simulink model "Final"  (R2025b)
settings: Solver=ode4  StartTime=0.0  StopTime=3  FixedStep=1e-5  RelTol=1e-3
values from neighbouring files (symbols this model uses):
  BAT_A = BAT    [simulink_init_params_CORRECTED.m]
  BAT_B = BAT    [simulink_init_params_CORRECTED.m]
  omega_init_cmd = SpeedRef_rpm_cmd * 2 * pi / 60    (= 314.159265359)    [simulink_init_params_CORRECTED.m]
  SpeedRef_rpm_cmd = 3000    [simulink_init_params_CORRECTED.m]
  TorqueRef_gen_Nm_cmd = -100    [simulink_init_params_CORRECTED.m]
undefined symbols (not defined in the file or in its folder): BAT, DCDC, DCLINK, FOC, FW, INV, MECH, PMSM, THERM
libraries: slpidlib x6, mcbcontrolslib x2
(part 2 of 2)

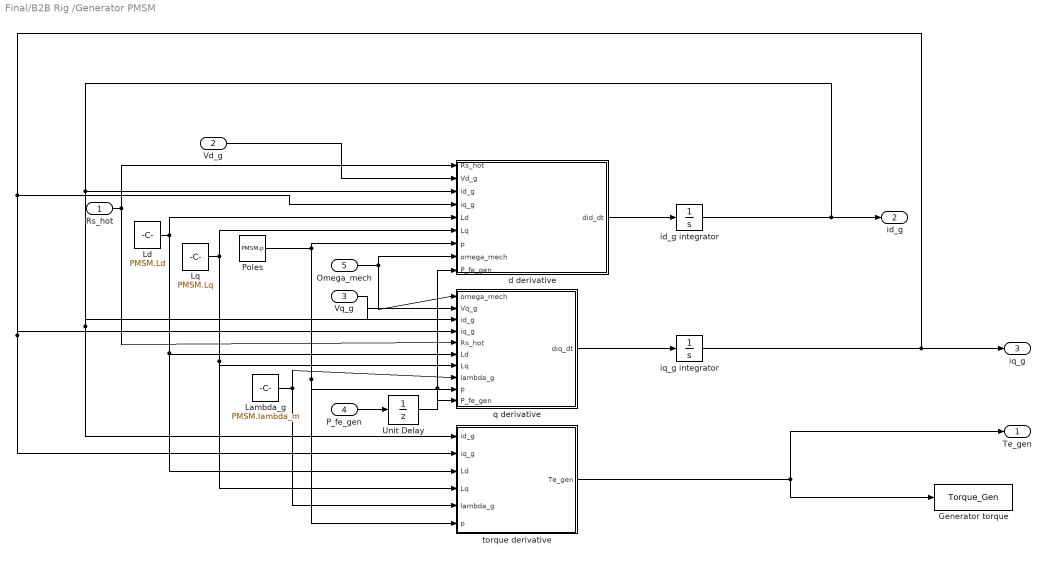
== system Final/B2B Rig /Generator PMSM ==
  Rs_hot : Inport
  Vd_g : Inport  Port=2
  Vq_g : Inport  Port=3
  P_fe_gen : Inport  Port=4
  Omega_mech : Inport  Port=5
  Generator torque : ToWorkspace  VariableName=Torque_Gen  SaveFormat=Timeseries  SampleTime=-1
  Lambda_g : Constant  Value=PMSM.lambda_m
  Ld : Constant  Value=PMSM.Ld
  Lq : Constant  Value=PMSM.Lq
  Poles : Constant  Value=PMSM.p
  Unit Delay : UnitDelay  SampleTime=FOC.Ts  HasFrameUpgradeWarning=on
  d derivative : MATLAB Function  TreatAsAtomicUnit=on
  id_g integrator : Integrator
  iq_g integrator : Integrator
  q derivative : MATLAB Function  TreatAsAtomicUnit=on
  torque derivative : MATLAB Function  TreatAsAtomicUnit=on
  Te_gen : Outport
  id_g : Outport  Port=2
  iq_g : Outport  Port=3
  wires:
  Lq/1 -> torque derivative/4(Lq), q derivative/7(Lq), d derivative/6(Lq)
  Poles/1 -> torque derivative/6(p), q derivative/9(p), d derivative/7(p)
  id_g integrator/1 -> id_g/1, d derivative/3(id_g), torque derivative/1(id_g), q derivative/3(id_g)
  Ld/1 -> torque derivative/3(Ld), q derivative/6(Ld), d derivative/5(Ld)
  iq_g integrator/1 -> iq_g/1, torque derivative/2(iq_g), q derivative/4(iq_g), d derivative/4(iq_g)
  Lambda_g/1 -> q derivative/8(lambda_g), torque derivative/5(lambda_g)
  Rs_hot/1 -> d derivative/1(Rs_hot), q derivative/5(Rs_hot)
  q derivative/1(diq_dt) -> iq_g integrator/1
  Omega_mech/1 -> q derivative/1(omega_mech), d derivative/8(omega_mech)
  Vq_g/1 -> q derivative/2(Vq_g)
  d derivative/1(did_dt) -> id_g integrator/1
  torque derivative/1(Te_gen) -> Generator torque/1, Te_gen/1
  Vd_g/1 -> d derivative/2(Vd_g)
  Unit Delay/1 -> d derivative/9(P_fe_gen), q derivative/10(P_fe_gen)
  P_fe_gen/1 -> Unit Delay/1

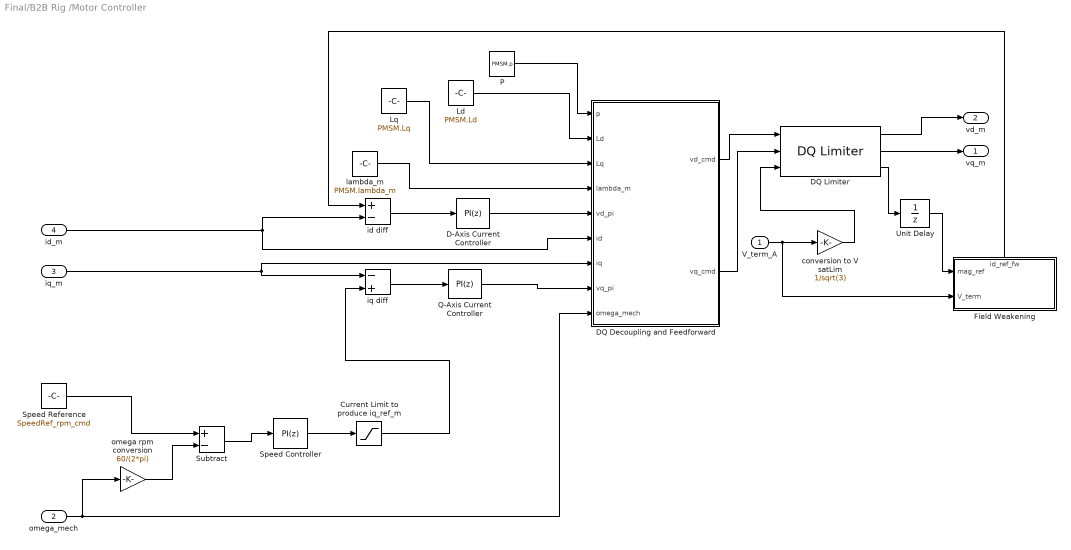
== system Final/B2B Rig /Motor Controller ==
  V_term_A : Inport
  omega_mech : Inport  Port=2
  iq_m : Inport  Port=3
  id_m : Inport  Port=4
  " Speed Controller" : slpidlib/PID Controller  Controller=PI  Form=Parallel  TimeDomain=Discrete-time  UseExternalTs=off  SampleTime=FOC.Ts  IntegratorMethod=Forward Euler  FilterMethod=Forward Euler  ControllerParametersSource=internal  P=FOC.Kp_speed  I=FOC.Ki_speed  UseKiTs=off  D=0  UseExternalDerivativeSource=off  N=100  UseFilter=on  TunerSelectOption=Transfer Function Based (PID Tuner App)  InitialConditionSource=internal  InitialConditionForIntegrator=0  InitialConditionForFilter=0  DifferentiatorICPrevScaledInput=0  ExternalReset=none  TrackingMode=off  Kt=1  LimitOutput=on  SatLimitsSource=internal  UpperSaturationLimit=FOC.I_limit  LowerSaturationLimit=-FOC.I_limit  LinearizeAsGain=on  AntiWindupMode=clamping  Kb=1  LimitIntegrator=off  UpperIntegratorSaturationLimit=inf  LowerIntegratorSaturationLimit=-inf  POutMin=[]  POutMax=[]  IOutMin=[]  IOutMax=[]  DOutMin=[]  DOutMax=[]  NOutMin=[]  NOutMax=[]  SumOutMin=[]  SumOutMax=[]  SaturationOutMin=[]  SaturationOutMax=[]  PParamMin=[]  PParamMax=[]  IParamMin=[]  IParamMax=[]  DParamMin=[]  DParamMax=[]  NParamMin=[]  NParamMax=[]  KbParamMin=[]  KbParamMax=[]  KtParamMin=[]  KtParamMax=[]  KbOutMin=[]  KbOutMax=[]  KtOutMin=[]  KtOutMax=[]  IntegratorOutMin=[]  IntegratorOutMax=[]  FilterOutMin=[]  FilterOutMax=[]  SumI1OutMin=[]  SumI1OutMax=[]  SumI2OutMin=[]  SumI2OutMax=[]  SumI3OutMin=[]  SumI3OutMax=[]  SumI4OutMin=[]  SumI4OutMax=[]  SumDOutMin=[]  SumDOutMax=[]  DifferentiatorOutMin=[]  DifferentiatorOutMax=[]  FilterDiffOutCoefMin=[]  FilterDiffOutCoefMax=[]  ReciprocalOutMin=[]  ReciprocalOutMax=[]  SumDenOutMin=[]  SumDenOutMax=[]  SumNumOutMin=[]  SumNumOutMax=[]  DivideOutMin=[]  DivideOutMax=[]  UdiffTsProdOutMin=[]  UdiffTsProdOutMax=[]  NTsProdOutMin=[]  NTsProdOutMax=[]  UintegralTsProdOutMin=[]  UintegralTsProdOutMax=[]  UngainTsProdOutMin=[]  UngainTsProdOutMax=[]  ClampingZeroOutDataTypeStr=Inherit: Inherit via back propagation  ClampingZeroOutMin=[]  ClampingZeroOutMax=[]  FilterDenConstantOutDataTypeStr=Inherit: Inherit via back propagation  FilterDenConstantOutMin=[]  FilterDenConstantOutMax=[]  PCopyOutDataTypeStr=Inherit: Inherit via back propagation  PCopyOutMin=[]  PCopyOutMax=[]  NCopyOutDataTypeStr=Inherit: Inherit via back propagation  NCopyOutMin=[]  NCopyOutMax=[]  IntegratorContinuousStateAttributes=''  IntegratorStateMustResolveToSignalObject=off  IntegratorRTWStateStorageClass=Auto  FilterContinuousStateAttributes=''  FilterStateMustResolveToSignalObject=off  FilterRTWStateStorageClass=Auto  ParallelPVariant=InternalParameters  IdealPVariant=Disabled  IVariant=InternalParameters  DVariant=Disabled  IntegratorVariant=Discrete  SatVariant=Enabled  AWVariant=DiscClampingParallel  PCopyVariant=Disabled  TRVariant=Disabled  FdbkBlocksVariant=Forward  IdealPFdbkVariant=Disabled  SatFdbkVariant=Disabled  DerivativeFilterVariant=Disabled  NVariant=Disabled  NCopyVariant=Disabled_SignalSpec  FilterICVariant=Disabled  IntegratorICVariant=InternalICs  ExternalResetVariant=Disabled  TRSumVariant=Passthrough  SumFdbkVariant=Disabled  SumVariant=Sum_PI  TsampFilterVariant=InternalTs  TsampNgainVariant=Passthrough  TsampIntegralVariant=Disabled_SignalSpec  ExternalSaturationOutDataTypeStr=Inherit: Same as second input  DerivativeSourceVariant=Disabled  PreIntVariant=InternalPreInt
  Current Limit to produce iq_ref_m : Saturate  UpperLimit=466.7  LowerLimit=-466.7
  D-Axis Current Controller : slpidlib/PID Controller  Controller=PI  Form=Parallel  TimeDomain=Discrete-time  UseExternalTs=off  SampleTime=FOC.Ts  IntegratorMethod=Forward Euler  FilterMethod=Forward Euler  ControllerParametersSource=internal  P=FOC.Kp_id  I=FOC.Ki_id  UseKiTs=off  D=0  UseExternalDerivativeSource=off  N=100  UseFilter=on  TunerSelectOption=Transfer Function Based (PID Tuner App)  InitialConditionSource=internal  InitialConditionForIntegrator=0  InitialConditionForFilter=0  DifferentiatorICPrevScaledInput=0  ExternalReset=none  TrackingMode=off  Kt=1  LimitOutput=on  SatLimitsSource=internal  UpperSaturationLimit=BAT.V_nom/sqrt(3)  LowerSaturationLimit=-BAT.V_nom/sqrt(3)  LinearizeAsGain=off  AntiWindupMode=clamping  Kb=1  LimitIntegrator=off  UpperIntegratorSaturationLimit=inf  LowerIntegratorSaturationLimit=-inf  POutMin=[]  POutMax=[]  IOutMin=[]  IOutMax=[]  DOutMin=[]  DOutMax=[]  NOutMin=[]  NOutMax=[]  SumOutMin=[]  SumOutMax=[]  SaturationOutMin=[]  SaturationOutMax=[]  PParamMin=[]  PParamMax=[]  IParamMin=[]  IParamMax=[]  DParamMin=[]  DParamMax=[]  NParamMin=[]  NParamMax=[]  KbParamMin=[]  KbParamMax=[]  KtParamMin=[]  KtParamMax=[]  KbOutMin=[]  KbOutMax=[]  KtOutMin=[]  KtOutMax=[]  IntegratorOutMin=[]  IntegratorOutMax=[]  FilterOutMin=[]  FilterOutMax=[]  SumI1OutMin=[]  SumI1OutMax=[]  SumI2OutMin=[]  SumI2OutMax=[]  SumI3OutMin=[]  SumI3OutMax=[]  SumI4OutMin=[]  SumI4OutMax=[]  SumDOutMin=[]  SumDOutMax=[]  DifferentiatorOutMin=[]  DifferentiatorOutMax=[]  FilterDiffOutCoefMin=[]  FilterDiffOutCoefMax=[]  ReciprocalOutMin=[]  ReciprocalOutMax=[]  SumDenOutMin=[]  SumDenOutMax=[]  SumNumOutMin=[]  SumNumOutMax=[]  DivideOutMin=[]  DivideOutMax=[]  UdiffTsProdOutMin=[]  UdiffTsProdOutMax=[]  NTsProdOutMin=[]  NTsProdOutMax=[]  UintegralTsProdOutMin=[]  UintegralTsProdOutMax=[]  UngainTsProdOutMin=[]  UngainTsProdOutMax=[]  ClampingZeroOutDataTypeStr=Inherit: Inherit via back propagation  ClampingZeroOutMin=[]  ClampingZeroOutMax=[]  FilterDenConstantOutDataTypeStr=Inherit: Inherit via back propagation  FilterDenConstantOutMin=[]  FilterDenConstantOutMax=[]  PCopyOutDataTypeStr=Inherit: Inherit via back propagation  PCopyOutMin=[]  PCopyOutMax=[]  NCopyOutDataTypeStr=Inherit: Inherit via back propagation  NCopyOutMin=[]  NCopyOutMax=[]  IntegratorContinuousStateAttributes=''  IntegratorStateMustResolveToSignalObject=off  IntegratorRTWStateStorageClass=Auto  FilterContinuousStateAttributes=''  FilterStateMustResolveToSignalObject=off  FilterRTWStateStorageClass=Auto  ParallelPVariant=InternalParameters  IdealPVariant=Disabled  IVariant=InternalParameters  DVariant=Disabled  IntegratorVariant=Discrete  SatVariant=Enabled  AWVariant=DiscClampingParallel  PCopyVariant=Disabled  TRVariant=Disabled  FdbkBlocksVariant=Forward  IdealPFdbkVariant=Disabled  SatFdbkVariant=Disabled  DerivativeFilterVariant=Disabled  NVariant=Disabled  NCopyVariant=Disabled_SignalSpec  FilterICVariant=Disabled  IntegratorICVariant=InternalICs  ExternalResetVariant=Disabled  TRSumVariant=Passthrough  SumFdbkVariant=Disabled  SumVariant=Sum_PI  TsampFilterVariant=InternalTs  TsampNgainVariant=Passthrough  TsampIntegralVariant=Disabled_SignalSpec  ExternalSaturationOutDataTypeStr=Inherit: Same as second input  DerivativeSourceVariant=Disabled  PreIntVariant=InternalPreInt
      settings: LibrarySourceBlock=simulink/Discrete/Discrete PID Controller
  DQ Decoupling and Feedforward : MATLAB Function  TreatAsAtomicUnit=on
  DQ Limiter : mcbcontrolslib/DQ Limiter  satMethodInputType=Specify via dialog  satMethodSelected=D-Q equivalence  satLimitInputType=Input port  Vmax=153
      settings: LibrarySourceBlock=mcblib/Controls/Control Reference/DQ Limiter
  Field Weakening : Subsystem
      settings: PortSchema="{\"entries\":[{\"content\":{\"sides\":[{\"content\":{\"connectorIds\":[\"In1\",\"In2\"]},\"type\":\"ConnectorPlacement.EquallySpacedRectSide\",\"uuid\":\"203a0201-c6d3-4021-9e02-f3e52e0315c3\"},{\"content\":{\"side\":\"RIGHT\"},\"type\":\"ConnectorPlacement.EquallySpacedRectSide\",\"uuid\":\"dc29f0d6-36ca-40be-93a9-96ff6b1d1e1c\"},{\"content\":{\"connectorIds\":[\"Out1\"],\"side\":\"TOP\"},\"type\":\"ConnectorPlacement.EquallySpacedRectSide\",\"uuid\":\"ca3e0a02-f9af-4c90-ae20-302966c67b10\"}]},\"type\":\"ConnectorPlacement.EquallySpacedConnector\",\"uuid\":\"9d944e2c-da2e-448a-8f6b-8a0454a994f1\"}],\"packageUris\":[\"http://schema.mathworks.com/mf0/Connector/R2020b\"],\"version\":\"1.0\"}"
  Ld : Constant  Value=PMSM.Ld
  Lq : Constant  Value=PMSM.Lq
  P : Constant  Value=PMSM.p
  Q-Axis Current Controller : slpidlib/PID Controller  Controller=PI  Form=Parallel  TimeDomain=Discrete-time  UseExternalTs=off  SampleTime=FOC.Ts  IntegratorMethod=Forward Euler  FilterMethod=Forward Euler  ControllerParametersSource=internal  P=FOC.Kp_iq  I=FOC.Ki_iq  UseKiTs=off  D=0  UseExternalDerivativeSource=off  N=100  UseFilter=on  TunerSelectOption=Transfer Function Based (PID Tuner App)  InitialConditionSource=internal  InitialConditionForIntegrator=0  InitialConditionForFilter=0  DifferentiatorICPrevScaledInput=0  ExternalReset=none  TrackingMode=off  Kt=1  LimitOutput=on  SatLimitsSource=internal  UpperSaturationLimit=BAT.V_nom/sqrt(3)  LowerSaturationLimit=-BAT.V_nom/sqrt(3)  LinearizeAsGain=off  AntiWindupMode=clamping  Kb=1  LimitIntegrator=off  UpperIntegratorSaturationLimit=inf  LowerIntegratorSaturationLimit=-inf  POutMin=[]  POutMax=[]  IOutMin=[]  IOutMax=[]  DOutMin=[]  DOutMax=[]  NOutMin=[]  NOutMax=[]  SumOutMin=[]  SumOutMax=[]  SaturationOutMin=[]  SaturationOutMax=[]  PParamMin=[]  PParamMax=[]  IParamMin=[]  IParamMax=[]  DParamMin=[]  DParamMax=[]  NParamMin=[]  NParamMax=[]  KbParamMin=[]  KbParamMax=[]  KtParamMin=[]  KtParamMax=[]  KbOutMin=[]  KbOutMax=[]  KtOutMin=[]  KtOutMax=[]  IntegratorOutMin=[]  IntegratorOutMax=[]  FilterOutMin=[]  FilterOutMax=[]  SumI1OutMin=[]  SumI1OutMax=[]  SumI2OutMin=[]  SumI2OutMax=[]  SumI3OutMin=[]  SumI3OutMax=[]  SumI4OutMin=[]  SumI4OutMax=[]  SumDOutMin=[]  SumDOutMax=[]  DifferentiatorOutMin=[]  DifferentiatorOutMax=[]  FilterDiffOutCoefMin=[]  FilterDiffOutCoefMax=[]  ReciprocalOutMin=[]  ReciprocalOutMax=[]  SumDenOutMin=[]  SumDenOutMax=[]  SumNumOutMin=[]  SumNumOutMax=[]  DivideOutMin=[]  DivideOutMax=[]  UdiffTsProdOutMin=[]  UdiffTsProdOutMax=[]  NTsProdOutMin=[]  NTsProdOutMax=[]  UintegralTsProdOutMin=[]  UintegralTsProdOutMax=[]  UngainTsProdOutMin=[]  UngainTsProdOutMax=[]  ClampingZeroOutDataTypeStr=Inherit: Inherit via back propagation  ClampingZeroOutMin=[]  ClampingZeroOutMax=[]  FilterDenConstantOutDataTypeStr=Inherit: Inherit via back propagation  FilterDenConstantOutMin=[]  FilterDenConstantOutMax=[]  PCopyOutDataTypeStr=Inherit: Inherit via back propagation  PCopyOutMin=[]  PCopyOutMax=[]  NCopyOutDataTypeStr=Inherit: Inherit via back propagation  NCopyOutMin=[]  NCopyOutMax=[]  IntegratorContinuousStateAttributes=''  IntegratorStateMustResolveToSignalObject=off  IntegratorRTWStateStorageClass=Auto  FilterContinuousStateAttributes=''  FilterStateMustResolveToSignalObject=off  FilterRTWStateStorageClass=Auto  ParallelPVariant=InternalParameters  IdealPVariant=Disabled  IVariant=InternalParameters  DVariant=Disabled  IntegratorVariant=Discrete  SatVariant=Enabled  AWVariant=DiscClampingParallel  PCopyVariant=Disabled  TRVariant=Disabled  FdbkBlocksVariant=Forward  IdealPFdbkVariant=Disabled  SatFdbkVariant=Disabled  DerivativeFilterVariant=Disabled  NVariant=Disabled  NCopyVariant=Disabled_SignalSpec  FilterICVariant=Disabled  IntegratorICVariant=InternalICs  ExternalResetVariant=Disabled  TRSumVariant=Passthrough  SumFdbkVariant=Disabled  SumVariant=Sum_PI  TsampFilterVariant=InternalTs  TsampNgainVariant=Passthrough  TsampIntegralVariant=Disabled_SignalSpec  ExternalSaturationOutDataTypeStr=Inherit: Same as second input  DerivativeSourceVariant=Disabled  PreIntVariant=InternalPreInt
      settings: LibrarySourceBlock=simulink/Discrete/Discrete PID Controller
  Speed Reference : Constant  Value=SpeedRef_rpm_cmd
  Subtract : Sum  Inputs=+-
  Unit Delay : UnitDelay  SampleTime=FOC.Ts  HasFrameUpgradeWarning=on
  conversion to V satLim : Gain  Gain=1/sqrt(3)
  id diff : Sum  Inputs=+-
  iq diff : Sum  Inputs=-+
  lambda_m : Constant  Value=PMSM.lambda_m
  omega rpm conversion : Gain  Gain=60/(2*pi)
  vq_m : Outport
  vd_m : Outport  Port=2
  wires:
  id_m/1 -> DQ Decoupling and Feedforward/6(id), id diff/2
  Speed Reference/1 -> Subtract/1
  Subtract/1 -> " Speed Controller"/1
  " Speed Controller"/1 -> Current Limit to produce iq_ref_m/1
  Current Limit to produce iq_ref_m/1 -> iq diff/2
  iq diff/1 -> Q-Axis Current Controller/1
  id diff/1 -> D-Axis Current Controller/1
  iq_m/1 -> DQ Decoupling and Feedforward/7(iq), iq diff/1
  Q-Axis Current Controller/1 -> DQ Decoupling and Feedforward/8(vq_pi)
  D-Axis Current Controller/1 -> DQ Decoupling and Feedforward/5(vd_pi)
  DQ Limiter/1 -> vd_m/1
  DQ Limiter/2 -> vq_m/1
  V_term_A/1 -> conversion to V satLim/1, Field Weakening/2(V_term)
  conversion to V satLim/1 -> DQ Limiter/3
  lambda_m/1 -> DQ Decoupling and Feedforward/4(lambda_m)
  Lq/1 -> DQ Decoupling and Feedforward/3(Lq)
  Ld/1 -> DQ Decoupling and Feedforward/2(Ld)
  P/1 -> DQ Decoupling and Feedforward/1(p)
  omega_mech/1 -> omega rpm conversion/1, DQ Decoupling and Feedforward/9(omega_mech)
  DQ Decoupling and Feedforward/2(vq_cmd) -> DQ Limiter/2
  DQ Decoupling and Feedforward/1(vd_cmd) -> DQ Limiter/1
  Field Weakening/1(id_ref_fw) -> id diff/1
  DQ Limiter/3 -> Unit Delay/1
  Unit Delay/1 -> Field Weakening/1(mag_ref)
  omega rpm conversion/1 -> Subtract/2

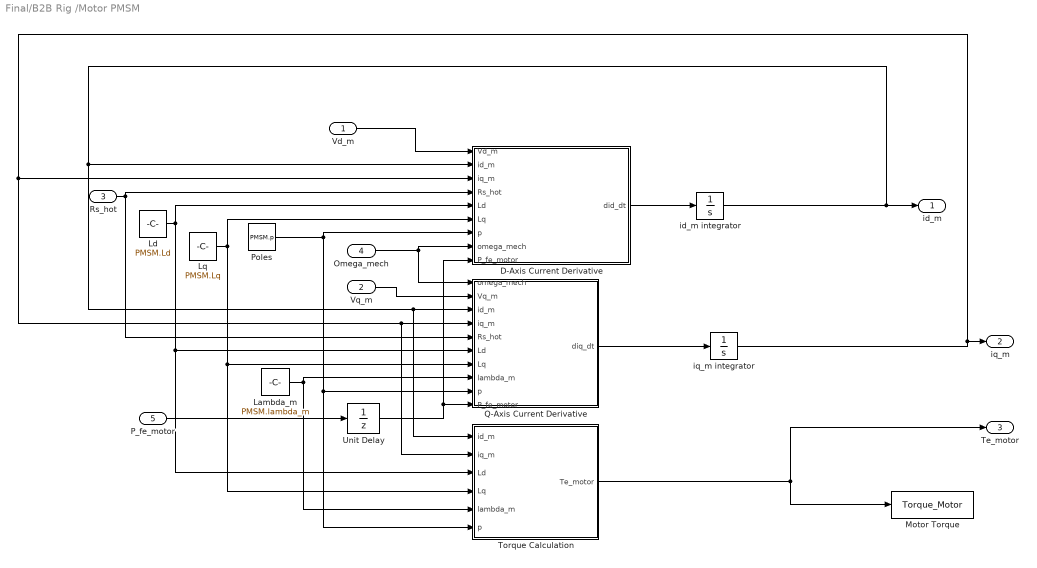
== system Final/B2B Rig /Motor PMSM ==
  Vd_m : Inport
  Vq_m : Inport  Port=2
  Rs_hot : Inport  Port=3
  Omega_mech : Inport  Port=4
  P_fe_motor : Inport  Port=5
  D-Axis Current Derivative : MATLAB Function  TreatAsAtomicUnit=on
  Lambda_m : Constant  Value=PMSM.lambda_m
  Ld : Constant  Value=PMSM.Ld
  Lq : Constant  Value=PMSM.Lq
  Motor Torque : ToWorkspace  VariableName=Torque_Motor  SaveFormat=Timeseries  SampleTime=-1
  Poles : Constant  Value=PMSM.p
  Q-Axis Current Derivative : MATLAB Function  TreatAsAtomicUnit=on
  Torque Calculation : MATLAB Function  TreatAsAtomicUnit=on
  Unit Delay : UnitDelay  SampleTime=FOC.Ts  HasFrameUpgradeWarning=on
  id_m integrator : Integrator
  iq_m integrator : Integrator
  id_m : Outport
  iq_m : Outport  Port=2
  Te_motor : Outport  Port=3
  wires:
  id_m integrator/1 -> Torque Calculation/1(id_m), Q-Axis Current Derivative/3(id_m), D-Axis Current Derivative/2(id_m), id_m/1
  iq_m integrator/1 -> Torque Calculation/2(iq_m), Q-Axis Current Derivative/4(iq_m), D-Axis Current Derivative/3(iq_m), iq_m/1
  Torque Calculation/1(Te_motor) -> Motor Torque/1, Te_motor/1
  Q-Axis Current Derivative/1(diq_dt) -> iq_m integrator/1
  D-Axis Current Derivative/1(did_dt) -> id_m integrator/1
  Vq_m/1 -> Q-Axis Current Derivative/2(Vq_m)
  Vd_m/1 -> D-Axis Current Derivative/1(Vd_m)
  Omega_mech/1 -> D-Axis Current Derivative/8(omega_mech), Q-Axis Current Derivative/1(omega_mech)
  Rs_hot/1 -> D-Axis Current Derivative/4(Rs_hot), Q-Axis Current Derivative/5(Rs_hot)
  Ld/1 -> Torque Calculation/3(Ld), Q-Axis Current Derivative/6(Ld), D-Axis Current Derivative/5(Ld)
  Lq/1 -> Q-Axis Current Derivative/7(Lq), Torque Calculation/4(Lq), D-Axis Current Derivative/6(Lq)
  Lambda_m/1 -> Torque Calculation/5(lambda_m), Q-Axis Current Derivative/8(lambda_m)
  Poles/1 -> Torque Calculation/6(p), Q-Axis Current Derivative/9(p), D-Axis Current Derivative/7(p)
  P_fe_motor/1 -> Unit Delay/1
  Unit Delay/1 -> Q-Axis Current Derivative/10(P_fe_motor), D-Axis Current Derivative/9(P_fe_motor)

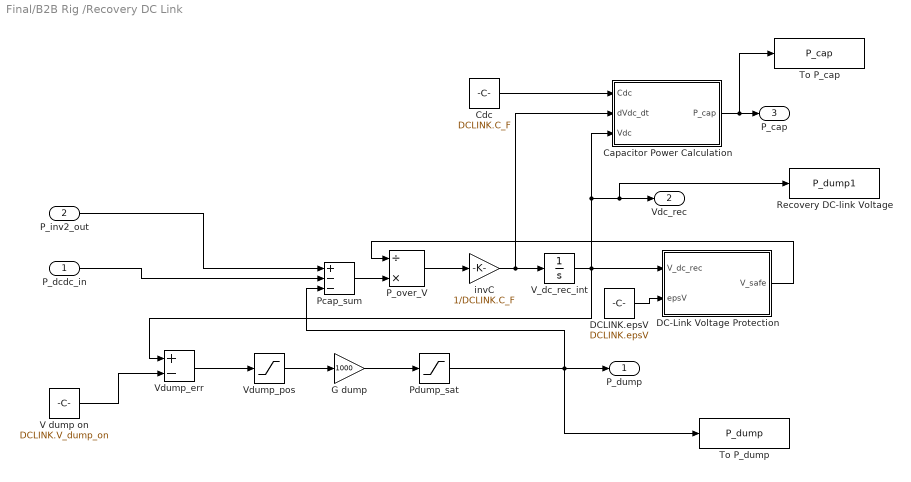
== system Final/B2B Rig /Recovery DC Link ==
  P_dcdc_in : Inport
  P_inv2_out : Inport  Port=2
  Capacitor Power Calculation : MATLAB Function  TreatAsAtomicUnit=on
  Cdc : Constant  Value=DCLINK.C_F
  DC-Link Voltage Protection : MATLAB Function  TreatAsAtomicUnit=on
  DCLINK.epsV : Constant  Value=DCLINK.epsV
  G dump : Gain  Gain=1000
  P_over_V : Product  Inputs=/*
  Pcap_sum : Sum  Inputs=+--
  Pdump_sat : Saturate  UpperLimit=DCLINK.P_dump_max  LowerLimit=0
  Recovery DC-link Voltage : ToWorkspace  VariableName=P_dump1  SaveFormat=Timeseries  SampleTime=-1
  To P_cap : ToWorkspace  VariableName=P_cap  SaveFormat=Timeseries  SampleTime=-1
  To P_dump : ToWorkspace  VariableName=P_dump  SaveFormat=Timeseries  SampleTime=-1
  "V dump on " : Constant  Value=DCLINK.V_dump_on
  V_dc_rec_int : Integrator  InitialCondition=DCLINK.V_init
  Vdump_err : Sum  Inputs=+-
  Vdump_pos : Saturate  UpperLimit=inf  LowerLimit=0
  invC : Gain  Gain=1/DCLINK.C_F
  P_dump : Outport
  Vdc_rec : Outport  Port=2
  P_cap : Outport  Port=3
  wires:
  P_inv2_out/1 -> Pcap_sum/1
  P_dcdc_in/1 -> Pcap_sum/2
  Vdump_err/1 -> Vdump_pos/1
  Vdump_pos/1 -> G dump/1
  G dump/1 -> Pdump_sat/1
  Pdump_sat/1 -> To P_dump/1, P_dump/1, Pcap_sum/3
  "V dump on "/1 -> Vdump_err/2
  V_dc_rec_int/1 -> Capacitor Power Calculation/3(Vdc), Recovery DC-link Voltage/1, Vdc_rec/1, DC-Link Voltage Protection/1(V_dc_rec), Vdump_err/1
  P_over_V/1 -> invC/1
  invC/1 -> Capacitor Power Calculation/2(dVdc_dt), V_dc_rec_int/1
  DC-Link Voltage Protection/1(V_safe) -> P_over_V/1
  Pcap_sum/1 -> P_over_V/2
  DCLINK.epsV/1 -> DC-Link Voltage Protection/2(epsV)
  Cdc/1 -> Capacitor Power Calculation/1(Cdc)
  Capacitor Power Calculation/1(P_cap) -> To P_cap/1, P_cap/1

== system Final/B2B Rig /Shaft Dynamics ==
  Te_motor : Inport
  Te_gen : Inport  Port=2
  1/MECH.J_total : Gain  Gain=1/MECH.J_total
  B_visc : Constant  Value=MECH.B_damping
  Motor/Generator Speed in RPM : ToWorkspace  VariableName=Speed_in_RPM  SaveFormat=Timeseries  SampleTime=-1
  Shaft Speed in RPM : Gain  Gain=60/(2*pi)
  T_f0 : Constant  Value=PMSM.mech.T_f0
  T_loss_mech : MATLAB Function  TreatAsAtomicUnit=on
  T_loss_visc : MATLAB Function  TreatAsAtomicUnit=on
  T_net : Sum  Inputs=++--
  k_w : Constant  Value=PMSM.mech.k_w
  omega mech int : Integrator  InitialCondition=omega_init_cmd
  omega_mech : Outport
  wires:
  T_net/1 -> 1/MECH.J_total/1
  1/MECH.J_total/1 -> omega mech int/1
  T_loss_visc/1(T_loss_visc) -> T_net/3
  T_loss_mech/1(T_loss_mech) -> T_net/4
  omega mech int/1 -> T_loss_mech/1(omega_mech), T_loss_visc/2(omega_mech), Shaft Speed in RPM/1, omega_mech/1
  B_visc/1 -> T_loss_visc/1(B_visc)
  T_f0/1 -> T_loss_mech/2(T_f0)
  k_w/1 -> T_loss_mech/3(k_w)
  Shaft Speed in RPM/1 -> Motor/Generator Speed in RPM/1
  Te_motor/1 -> T_net/2
  Te_gen/1 -> T_net/1

== system Final/B2B Rig /Winding Thermal ==
  P_cu : Inport
  " Windage temp" : ToWorkspace  VariableName=T_wind  SaveFormat=Timeseries  SampleTime=-1
  Cth_wind : Constant  Value=THERM.Cth_wind
  Rs_hot Calculation : MATLAB Function  TreatAsAtomicUnit=on
  Rs_ref : Constant  Value=THERM.Rs_ref
  Rth_wind : Constant  Value=THERM.Rth_wind
  T_amb : Constant  Value=THERM.T_amb
  T_ref : Constant  Value=THERM.T_ref
  T_wind Integrator : Integrator  InitialCondition=THERM.T_init
  alpha_cu : Constant  Value=THERM.alpha_cu
  dT_dt Calculation : MATLAB Function  TreatAsAtomicUnit=on
  Rs_hot : Outport
  wires:
  T_wind Integrator/1 -> dT_dt Calculation/1(T_wind), " Windage temp"/1, Rs_hot Calculation/1(T_wind)
  dT_dt Calculation/1(dT_dt) -> T_wind Integrator/1
  Rs_hot Calculation/1(Rs_hot) -> Rs_hot/1
  P_cu/1 -> dT_dt Calculation/2(P_cu)
  T_amb/1 -> dT_dt Calculation/3(T_amb)
  Rth_wind/1 -> dT_dt Calculation/4(Rth_wind)
  Cth_wind/1 -> dT_dt Calculation/5(Cth_wind)
  Rs_ref/1 -> Rs_hot Calculation/2(Rs_ref)
  alpha_cu/1 -> Rs_hot Calculation/3(alpha_cu)
  T_ref/1 -> Rs_hot Calculation/4(T_ref)

== system Final/B2B Rig /Generator Controller/Field Weakening ==
  mag_ref : Inport
  V_term : Inport  Port=2
  " Field Weakening" : MATLAB Function  TreatAsAtomicUnit=on
  K_fw : Constant  Value=FW.k_fw
  id_min : Constant  Value=FW.id_min
  k_trigger : Constant  Value=FW.k_trigger
  id_ref_fw : Outport
  wires:
  " Field Weakening"/1(id_ref_fw) -> id_ref_fw/1
  mag_ref/1 -> " Field Weakening"/1(mag_ref)
  V_term/1 -> " Field Weakening"/2(V_term)
  k_trigger/1 -> " Field Weakening"/3(k_trigger)
  K_fw/1 -> " Field Weakening"/4(K_fw)
  id_min/1 -> " Field Weakening"/5(id_min)

== system Final/B2B Rig /Motor Controller/Field Weakening ==
  mag_ref : Inport
  V_term : Inport  Port=2
  " Field Weakening" : MATLAB Function  TreatAsAtomicUnit=on
  K_fw : Constant  Value=FW.k_fw
  id_min : Constant  Value=FW.id_min
  k_trigger : Constant  Value=FW.k_trigger
  id_ref_fw : Outport
  wires:
  " Field Weakening"/1(id_ref_fw) -> id_ref_fw/1
  mag_ref/1 -> " Field Weakening"/1(mag_ref)
  V_term/1 -> " Field Weakening"/2(V_term)
  k_trigger/1 -> " Field Weakening"/3(k_trigger)
  K_fw/1 -> " Field Weakening"/4(K_fw)
  id_min/1 -> " Field Weakening"/5(id_min)

== matlab function Final/B2B Rig /Battery A DC Bus/Battery A ==
  data: V_term_A output; P_bat_loss_A output; I_batt_A output; P_battA_max output; dSOC_dt output; P_req_motor_dc input; V_max input; V_min input; R_int input; C_Ah input; SOC_A input
function [V_term_A, P_bat_loss_A, I_batt_A, P_battA_max, dSOC_dt] = BatteryA( ...
    P_req_motor_dc, V_max, V_min, R_int, C_Ah, SOC_A)

% Source battery only
% Positive current = discharge

V_oc = V_min + (V_max - V_min) * SOC_A;

P_req = max(P_req_motor_dc, 0);

% Maximum terminal power of Thevenin source
if R_int > 1e-9
    P_battA_max = V_oc^2 / (4*R_int);
else
    P_battA_max = inf;
end

% Enforce physical max power
P_req = min(P_req, P_battA_max);

% Solve R*I^2 - V_oc*I + P_req = 0
if R_int > 1e-9
    disc = V_oc^2 - 4*R_int*P_req;
    disc = max(disc, 0);
    I_batt_A = (V_oc - sqrt(disc)) / (2*R_int);
else
    if V_oc > 1e-9
        I_batt_A = P_req / V_oc;
    else
        I_batt_A = 0;
    end
end

I_batt_A = max(I_batt_A, 0);

V_term_A      = V_oc - I_batt_A*R_int;
P_bat_loss_A  = I_batt_A^2 * R_int;
dSOC_dt       = -I_batt_A / (C_Ah * 3600);
end

== matlab function Final/B2B Rig /Motor Controller/DQ Decoupling and Feedforward ==
  data: p input; Ld input; Lq input; lambda_m input; vd_pi input; id input; iq input; vd_cmd output; vq_pi input; omega_mech input; vq_cmd output
function [vd_cmd, vq_cmd] = fcn(p, Ld, Lq, lambda_m, vd_pi, id, iq, vq_pi, omega_mech)

omega_e = p * omega_mech;

vd_ff = -omega_e * Lq * iq;
vq_ff =  omega_e * (Ld * id + lambda_m);

vd_cmd = vd_pi + vd_ff;
vq_cmd = vq_pi + vq_ff;

== matlab function Final/B2B Rig /Generator Controller/DQ Decoupling//Feedforward ==
  data: p input; Ld input; Lq input; lambda_m input; vd_pi input; id input; iq input; vd_cmd output; vq_pi input; omega_mech input; vq_cmd output
function [vd_cmd, vq_cmd] = fcn(p, Ld, Lq, lambda_m, vd_pi, id, iq, vq_pi, omega_mech)

omega_e = p * omega_mech;

vd_ff = -omega_e * Lq * iq;
vq_ff =  omega_e * (Ld * id + lambda_m);

vd_cmd = vd_pi + vd_ff;
vq_cmd = vq_pi + vq_ff;

== matlab function Final/Loss Calculator/Copper Loss Calculation ==
  data: iq_m input; id_m input; Rs_hot input; P_cu_motor output; id_g input; iq_g input; P_cu_gen output; P_cu_total output
function [P_cu_motor, P_cu_gen, P_cu_total] = fcn(iq_m,id_m,Rs_hot,id_g,iq_g)
% Copper losses split by machine

Irm_m = sqrt(id_m.^2 + iq_m.^2) / sqrt(2);
Irm_g = sqrt(id_g.^2 + iq_g.^2) / sqrt(2);

P_cu_motor = 3 * Rs_hot * Irm_m.^2;
P_cu_gen   = 3 * Rs_hot * Irm_g.^2;
P_cu_total = P_cu_motor + P_cu_gen;
end

== matlab function Final/Loss Calculator/Iron Loss Calculation ==
  data: omega_mech input; P_fe_motor output; p input; k_h input; k_e input; alpha input; B_pk input; P_fe_gen output; P_fe_total output
function [P_fe_motor, P_fe_gen, P_fe_total] = fcn(omega_mech,p,k_h,k_e,alpha,B_pk)
% Core / iron losses split by machine

f_e = p * abs(omega_mech) / (2*pi);

P_fe_one = k_h * (f_e.^alpha) + k_e * (f_e * B_pk).^2;

% Identical machines on the same shaft speed
P_fe_motor = P_fe_one;
P_fe_gen   = P_fe_one;
P_fe_total = P_fe_motor + P_fe_gen;
end

== matlab function Final/Loss Calculator/Mechanical Loss Calculation ==
  data: T_f0 input; k_w input; omega_mech input; P_mech_loss output; B_damping input
function P_mech_loss = fcn(T_f0,k_w,omega_mech, B_damping)
%Friction + windage + viscous damping losses

w = abs(omega_mech);

P_mech_loss = T_f0*w + k_w*w.^3+B_damping*w.^2;
end

== matlab function Final/Loss Calculator/Inverter 1 Loss Calculation ==
  data: V_CE_sat input; V_D_fwd input; E_on input; E_off input; f_sw input; V_dc input; id_m input; P_inv1 output; iq_m input
function P_inv1 = fcn(V_CE_sat,V_D_fwd,E_on,E_off,f_sw,V_dc,id_m,iq_m)
% Motor-side inverter loss

Irm = sqrt(id_m^2 + iq_m^2) / sqrt(2);

P_cond = 3 * Irm * (V_CE_sat + V_D_fwd) * (2/3);
P_sw   = (E_on + E_off) * Irm * V_dc * f_sw;

P_inv1 = P_cond + P_sw;
end

== matlab function Final/Loss Calculator/Inverter 2 Loss Calculation ==
  data: iq_g input; id_g input; V_dc input; f_sw input; E_off input; E_on input; V_D_fwd input; P_inv2 output; V_CE_sat input
function P_inv2 = fcn(iq_g,id_g,V_dc,f_sw,E_off,E_on,V_D_fwd,V_CE_sat)
% Generator-side inverter loss

Irm = sqrt(id_g^2 + iq_g^2) / sqrt(2);

P_cond = 3*Irm*(V_CE_sat + V_D_fwd)*(2/3);
P_sw   = (E_on + E_off)*Irm*V_dc*f_sw;

P_inv2 = P_cond + P_sw;
end

== matlab function Final/B2B Rig /Generator PMSM/d derivative ==
  data: Rs_hot input; Vd_g input; did_dt output; id_g input; iq_g input; Ld input; Lq input; p input; omega_mech input; P_fe_gen input
function did_dt = fcn(Rs_hot,Vd_g,id_g,iq_g,Ld,Lq,p,omega_mech,P_fe_gen)

omega_e = p * omega_mech;

% Iron loss as equivalent series resistance
I_sq = id_g^2 + iq_g^2;
Rc_eq = P_fe_gen * 2 / max(3 * I_sq, 1e-3);
Rc_eq = min(Rc_eq, 10*Rs_hot);
Rs_tot = Rs_hot + Rc_eq;

did_dt = (Vd_g - Rs_tot*id_g + omega_e*Lq*iq_g) / Ld;
end

== matlab function Final/B2B Rig /Generator PMSM/q derivative ==
  data: omega_mech input; Vq_g input; diq_dt output; id_g input; iq_g input; Rs_hot input; Ld input; Lq input; lambda_g input; p input; P_fe_gen input
function diq_dt = fcn(omega_mech,Vq_g,id_g,iq_g,Rs_hot,Ld,Lq,lambda_g,p,P_fe_gen)

omega_e = p * omega_mech;

% Iron loss as equivalent series resistance
I_sq = id_g^2 + iq_g^2;
Rc_eq = P_fe_gen * 2 / max(3 * I_sq, 1e-3);
Rc_eq = min(Rc_eq, 10*Rs_hot);
Rs_tot = Rs_hot + Rc_eq;

diq_dt = (Vq_g - Rs_tot*iq_g - omega_e*(Ld*id_g + lambda_g)) / Lq;
end

== matlab function Final/B2B Rig /Generator PMSM/torque derivative ==
  data: id_g input; Te_gen output; iq_g input; Ld input; Lq input; lambda_g input; p input
function Te_gen = fcn(id_g,iq_g,Ld,Lq,lambda_g,p)

Te_gen = 1.5*p*(lambda_g*iq_g + (Ld - Lq)*id_g*iq_g);

== matlab function Final/Power Calculator/Battery A Power  ==
  data: V_term_A input; P_battA_out output; I_batt_A input
function P_battA_out = fcn(V_term_A,I_batt_A)
% Battery A output power to motor-side inverter/DC bus

P_battA_out = V_term_A .* I_batt_A;

end

== matlab function Final/B2B Rig /Winding Thermal/dT_dt Calculation ==
  data: T_wind input; P_cu input; dT_dt output; T_amb input; Rth_wind input; Cth_wind input
function dT_dt  = fcn( T_wind, P_cu,T_amb, Rth_wind, Cth_wind)

% Thermal dynamics
dT_dt = (P_cu - (T_wind - T_amb)/Rth_wind) / Cth_wind;

end

== matlab function Final/B2B Rig /Generator Controller/Field Weakening/ Field Weakening ==
  data: mag_ref input; id_ref_fw output; V_term input; k_trigger input; K_fw input; id_min input
function id_ref_fw = fcn(mag_ref, V_term, k_trigger, K_fw, id_min)

Vmax = V_term / sqrt(3);
e_fw = mag_ref - k_trigger * Vmax;

if e_fw <= 0
    id_ref_fw = 0;
else
    id_ref_fw = -K_fw * e_fw;
end

if id_ref_fw < id_min
    id_ref_fw = id_min;
end

== matlab function Final/B2B Rig /Motor Controller/Field Weakening/ Field Weakening ==
  data: mag_ref input; id_ref_fw output; V_term input; k_trigger input; K_fw input; id_min input
function id_ref_fw = fcn(mag_ref, V_term, k_trigger, K_fw, id_min)

Vmax = V_term / sqrt(3);
e_fw = mag_ref - k_trigger * Vmax;

if e_fw <= 0
    id_ref_fw = 0;
else
    id_ref_fw = -K_fw * e_fw;
end

if id_ref_fw < id_min
    id_ref_fw = id_min;
end

== matlab function Final/B2B Rig /Winding Thermal/Rs_hot Calculation ==
  data: T_wind input; Rs_ref input; alpha_cu input; T_ref input; Rs_hot output
function Rs_hot = fcn(T_wind, Rs_ref, alpha_cu, T_ref)

% Equation for Rs_hot
Rs_hot = Rs_ref * (1 + alpha_cu * (T_wind - T_ref));

if Rs_hot < 0
    Rs_hot = Rs_ref;
end

== matlab function Final/B2B Rig /Battery B DC Bus/Battery B ==
  data: V_term_B output; P_bat_loss output; I_batt_B output; P_charge_dc input; V_max input; V_min input; R_int input; C_Ah input; I_charge_max input; SOC_B input; dSOC_dt output
function [V_term_B, P_bat_loss, I_batt_B, dSOC_dt] = BatteryB( ...
    P_charge_dc, V_max, V_min, R_int, C_Ah, I_charge_max, SOC_B)

% Battery B = sink battery only
% Positive current = charge into Battery B
% P_charge_dc is charger power delivered to battery terminals

V_oc = V_min + (V_max - V_min) * SOC_B;
P_charge_dc = max(P_charge_dc, 0);

% Solve terminal power equation:
% P_charge_dc = V_term_B * I = (V_oc + I*R_int) * I
% => R_int*I^2 + V_oc*I - P_charge_dc = 0

if R_int > 1e-9
    disc = V_oc^2 + 4*R_int*P_charge_dc;
    I_batt_B = (-V_oc + sqrt(max(disc,0))) / (2*R_int);
else
    if V_oc > 1e-9
        I_batt_B = P_charge_dc / V_oc;
    else
        I_batt_B = 0;
    end
end

I_batt_B = min(max(I_batt_B, 0), abs(I_charge_max));

V_term_B      = V_oc + I_batt_B * R_int;
P_bat_loss    = I_batt_B^2 * R_int;

dSOC_dt = I_batt_B / (C_Ah * 3600);
end

== matlab function Final/B2B Rig /Recovery DC Link/DC-Link Voltage Protection ==
  data: V_dc_rec input; V_safe output; epsV input
function V_safe = safeV(V_dc_rec, epsV)
V_safe = max(V_dc_rec, epsV);

== matlab function Final/Power Calculator/Inverter 1 Power ==
  data: P_battA_out input; P_inv1_out output; P_inv1_loss input
function P_inv1_out = fcn(P_battA_out, P_inv1_loss)
% Generator inverter DC-side output power
% Use AC-side generator electrical power minus inverter loss

PbattA_out = abs(P_battA_out);
Pinv1_loss    = abs(P_inv1_loss);

P_inv1_out = max(PbattA_out - Pinv1_loss, 0);
end

== matlab function Final/Power Calculator/Motor Electrical Power ==
  data: vd_m input; P_motor_elec_in output; vq_m input; id_m input; iq_m input
function P_motor_elec_in = fcn(vd_m,vq_m,id_m,iq_m)
% Motor electrical input power in dq frame

P_motor_elec_in = 1.5 * (vd_m .* id_m + vq_m .* iq_m);
end

== matlab function Final/B2B Rig /Averaged Bidirectional DC-DC Converter/Battery Voltage Protection ==
  data: epsV input; V_term_B input; V_safe output
function V_safe = safeVbatt(epsV, V_term_B)
V_safe = max(V_term_B, epsV);

== matlab function Final/B2B Rig /Charge Supervisor/Rotor Speed Protection ==
  data: omega input; omega_safe output; n_max input
function omega_safe = fcn(omega,n_max)
%#codegen
% Limits rotor speed magnitude to avoid numerical instability and prevent
% speeds above the PMSM maximum speed.

omega_min = 1;                       % rad/s
omega_max = n_max * 2*pi / 60;       % 6500 rpm converted to rad/s

omega_abs = abs(omega);

omega_safe = min(max(omega_abs, omega_min), omega_max);

end

== matlab function Final/Efficiency Calculator/Efficiency Split Calculation ==
  data: eta_battA output; P_battA_out input; P_inv1_out input; P_motor_mech_out input; P_gen_mech_in input; P_gen_elec_out input; P_inv2_out input; P_dcdc_in input; P_dcdc_out input; P_battB_in input; P_bat_loss_A input; P_bat_loss_B input; eta_inv1 output; P_cu_motor input; eta_motor output; eta_shaft output; eta_gen output; eta_inv2 output; eta_dcdc output; eta_battB output; eta_regen output; eta_rig output; eta_b2b output; P_fe_motor input; P_cu_gen input; P_fe_gen input; motor_balance_W output; gen_balance_W output
function [eta_battA, eta_inv1, eta_motor, eta_shaft, ...
          eta_gen, eta_inv2, eta_dcdc, eta_battB, ...
          eta_regen, eta_rig, eta_b2b, ...
          motor_balance_W, gen_balance_W] = ...
    fcn(P_battA_out, P_inv1_out, ...
        P_motor_mech_out, P_gen_mech_in, P_gen_elec_out, ...
        P_inv2_out, P_dcdc_in, P_dcdc_out, ...
        P_battB_in, P_bat_loss_A, P_bat_loss_B, ...
        P_cu_motor, P_fe_motor, P_cu_gen, P_fe_gen)
%#codegen
%
% CONSISTENT MACHINE EFFICIENCY DEFINITIONS
%
% Motor:
%   eta_motor = P_motor_mech_out / (P_motor_mech_out + P_cu_motor + P_fe_motor)
%
% Generator:
%   eta_gen   = P_gen_elec_out   / (P_gen_elec_out   + P_cu_gen   + P_fe_gen)
%
% Shaft loss is excluded from both machine efficiencies and handled separately:
%   eta_shaft = P_gen_mech_in / P_motor_mech_out
%
% Battery-B convention:
%   P_dcdc_out = Battery-B terminal charging power
%   P_battB_in = Battery-B stored power
%   P_bat_loss_B = Battery-B internal charging loss
%
% So:
%   P_battB_term = P_dcdc_out
%
% Notes:
% - This makes motor and generator efficiencies directly comparable.
% - The optional outputs motor_balance_W and gen_balance_W are useful
%   diagnostics to verify that the logged stage powers match the split losses.

eps_val = 1e-6;

% Forward-power conventions
P_battA_fwd      = max(P_battA_out,      0);
P_inv1_fwd       = max(P_inv1_out,       0);
P_motor_mech_fwd = max(P_motor_mech_out, 0);

P_gen_mech_fwd   = max(-P_gen_mech_in,  0);
P_gen_elec_fwd   = max(-P_gen_elec_out,  0);

P_inv2_fwd       = max(P_inv2_out,       0);
P_dcdc_in_fwd    = max(P_dcdc_in,        0);
P_dcdc_out_fwd   = max(P_dcdc_out,       0);

P_battB_store_fwd = max(P_battB_in, 0);
P_battB_term_fwd  = P_dcdc_out_fwd;

P_bat_loss_A_pos = max(P_bat_loss_A, 0);
P_bat_loss_B_pos = max(P_bat_loss_B, 0);

P_cu_motor_fwd = max(P_cu_motor, 0);
P_fe_motor_fwd = max(P_fe_motor, 0);
P_cu_gen_fwd   = max(P_cu_gen,   0);
P_fe_gen_fwd   = max(P_fe_gen,   0);

% Reconstructed comparable machine input/output balances
P_motor_elec_bal = P_motor_mech_fwd + P_cu_motor_fwd + P_fe_motor_fwd;
P_gen_mech_bal   = P_gen_elec_fwd   + P_cu_gen_fwd   + P_fe_gen_fwd;

% Diagnostics
motor_balance_W = P_inv1_fwd    - P_motor_elec_bal;
gen_balance_W   = P_gen_mech_fwd - P_gen_mech_bal;

% Stage efficiencies
eta_battA = P_battA_fwd / max(P_battA_fwd + P_bat_loss_A_pos, eps_val);
eta_inv1  = P_inv1_fwd  / max(P_battA_fwd, eps_val);

eta_motor = P_motor_mech_fwd / max(P_motor_elec_bal, eps_val);
eta_shaft = P_gen_mech_fwd   / max(P_motor_mech_fwd, eps_val);
eta_gen   = P_gen_elec_fwd   / max(P_gen_mech_bal, eps_val);

eta_inv2  = P_inv2_fwd      / max(P_gen_elec_fwd, eps_val);
eta_dcdc  = P_dcdc_out_fwd  / max(P_dcdc_in_fwd, eps_val);
eta_battB = P_battB_store_fwd / max(P_battB_term_fwd, eps_val);

eta_regen = P_battB_store_fwd / max(P_gen_mech_fwd, eps_val);
eta_rig   = P_battB_store_fwd / max(P_battA_fwd, eps_val);
eta_b2b   = P_battB_term_fwd  / max(P_battA_fwd, eps_val);

% Clamp to [0,1]
eta_battA = min(max(eta_battA,0),1);
eta_inv1  = min(max(eta_inv1 ,0),1);
eta_motor = min(max(eta_motor,0),1);
eta_shaft = min(max(eta_shaft,0),1);
eta_gen   = min(max(eta_gen  ,0),1);
eta_inv2  = min(max(eta_inv2 ,0),1);
eta_dcdc  = min(max(eta_dcdc ,0),1);
eta_battB = min(max(eta_battB,0),1);
eta_regen = min(max(eta_regen,0),1);
eta_rig   = min(max(eta_rig  ,0),1);
eta_b2b   = min(max(eta_b2b  ,0),1);
end

== matlab function Final/Power Calculator/Generator Electric Power ==
  data: vd_g input; P_gen_elec_out output; vq_g input; id_g input; iq_g input
function P_gen_elec_out = fcn(vd_g,vq_g,id_g,iq_g)
% Generator electrical output power in dq frame

P_gen_elec_out = 1.5 * (vd_g .* id_g + vq_g .* iq_g);
end

== matlab function Final/B2B Rig /Shaft Dynamics/T_loss_visc ==
  data: T_loss_visc output; B_visc input; omega_mech input
function T_loss_visc = fcn(B_visc,omega_mech)

T_loss_visc = B_visc * omega_mech;

== matlab function Final/Power Calculator/Motor Mechanical Power ==
  data: Te_motor input; P_motor_mech_out output; omega_mech input
function P_motor_mech_out = fcn(Te_motor,omega_mech)
% Motor mechanical output power

P_motor_mech_out = Te_motor .* omega_mech;
end

== matlab function Final/B2B Rig /Recovery DC Link/Capacitor Power Calculation ==
  data: Cdc input; dVdc_dt input; Vdc input; P_cap output
function P_cap = fcn(Cdc, dVdc_dt,Vdc)
% DC-link capacitor power
P_cap = Cdc .* Vdc .* dVdc_dt;
end

== matlab function Final/Power Calculator/Generator Mechanical Power ==
  data: Te_gen input; omega_mech input; P_gen_mech_in output
function P_gen_mech_in = fcn(Te_gen,omega_mech)
% Generator mechanical input power

P_gen_mech_in = Te_gen .* omega_mech;
end

== matlab function Final/Power Calculator/Inverter 2 Power ==
  data: P_gen_elec_out input; P_inv2_out output; P_inv2_loss input
function P_inv2_out = fcn(P_gen_elec_out, P_inv2_loss)
% Actual inverter-2 DC-side output power into recovered DC link
P_inv2_out = abs(P_gen_elec_out)-P_inv2_loss;
end

== matlab function Final/Power Calculator/DCDC Input Power ==
  data: eta_chg input; P_dcdc_out input; P_dcdc_in output
function P_dcdc_in = fcn(eta_chg, P_dcdc_out)
% Actual DC/DC input power drawn from recovered DC link
eta = max(eta_chg, 1e-6);
P_dcdc_in = max(P_dcdc_out, 0) / eta;
end

== matlab function Final/Power Calculator/DCDC Output Power ==
  data: V_term_B input; I_batt_B input; P_dcdc_out output
function P_dcdc_out = fcn(V_term_B, I_batt_B)
% Actual DC/DC output power delivered to Battery B terminals
P_dcdc_out = V_term_B .* I_batt_B;
end

== matlab function Final/Power Calculator/Battery B Powered Stored ==
  data: P_dcdc_out input; P_bat_loss_B input; P_battB_in output; P_dump input; P_cap input
function P_battB_in = fcn(P_dcdc_out,P_bat_loss_B,P_dump,P_cap)
% Battery B charging power

P_battB_in = P_dcdc_out - (P_bat_loss_B + P_dump + P_cap);
end

== matlab function Final/B2B Rig /Inverter 2 Output Power Calculation ==
  data: P_gen_elec_out input; P_inv2_loss input; P_inv2_out output
function P_inv2_out = fcn(P_gen_elec_out,P_inv2_loss)

P_inv2_out = P_gen_elec_out - P_inv2_loss;
end

== matlab function Final/B2B Rig /Motor DC Power Request Calculation ==
  data: id_m input; P_req_motor_dc output; iq_m input; vd_m input; vq_m input; P_inv1_loss input
function P_req_motor_dc = fcn(id_m, iq_m, vd_m, vq_m, P_inv1_loss)
P_req_motor_dc = 1.5 * (vd_m*id_m + vq_m*iq_m) + P_inv1_loss;
end

== matlab function Final/B2B Rig /Shaft Dynamics/T_loss_mech ==
  data: omega_mech input; T_loss_mech output; T_f0 input; k_w input
function T_loss_mech = fcn(omega_mech,T_f0,k_w)

if abs(omega_mech) < 1e-6
    T_loss_mech = 0;
else
    T_loss_mech = sign(omega_mech) * (T_f0 + k_w * omega_mech.^2);
end

== matlab function Final/B2B Rig /Generator Electrical Power Calculation ==
  data: id_g input; iq_g input; vd_g input; P_gen_elec_out output; vq_g input
function P_gen_elec_out = fcn(id_g,iq_g,vd_g,vq_g)

P_gen_elec_out = 1.5 * (vd_g*id_g + vq_g*iq_g);
end

== matlab function Final/B2B Rig /DQ Voltage Calculation ==
  data: V_term_A input; vq_cmd input; vd_cmd input; vd_act output; vq_act output
function [vd_act, vq_act] = fcn( V_term_A, vq_cmd, vd_cmd)
Vmax = V_term_A / sqrt(3);
mag = sqrt(vd_cmd^2 + vq_cmd^2);

if mag > Vmax && mag > 1e-9
    s = Vmax / mag;
else
    s = 1;
end

vd_act = vd_cmd * s;
vq_act = vq_cmd * s;
end

== matlab function Final/B2B Rig /Motor PMSM/D-Axis Current Derivative ==
  data: Vd_m input; did_dt output; id_m input; iq_m input; Rs_hot input; Ld input; Lq input; p input; omega_mech input; P_fe_motor input
function did_dt = fcn(Vd_m,id_m,iq_m,Rs_hot,Ld,Lq,p,omega_mech,P_fe_motor)

omega_e = p * omega_mech;

% Iron loss as equivalent series resistance
I_sq = id_m^2 + iq_m^2;
Rc_eq = P_fe_motor * 2 / max(3 * I_sq, 1e-3);
Rc_eq = min(Rc_eq, 10*Rs_hot);
Rs_tot = Rs_hot + Rc_eq;

did_dt = (Vd_m - Rs_tot*id_m + omega_e*Lq*iq_m) / Ld;

== matlab function Final/B2B Rig /Motor PMSM/Q-Axis Current Derivative ==
  data: omega_mech input; Vq_m input; diq_dt output; id_m input; iq_m input; Rs_hot input; Ld input; Lq input; lambda_m input; p input; P_fe_motor input
function diq_dt = fcn(omega_mech,Vq_m,id_m,iq_m,Rs_hot,Ld,Lq,lambda_m,p,P_fe_motor)

omega_e = p * omega_mech;

% Iron loss as equivalent series resistance
I_sq = id_m^2 + iq_m^2;
Rc_eq = P_fe_motor * 2 / max(3 * I_sq, 1e-3);
Rc_eq = min(Rc_eq, 10*Rs_hot);
Rs_tot = Rs_hot + Rc_eq;

diq_dt = (Vq_m - Rs_tot*iq_m - omega_e*(Ld*id_m + lambda_m)) / Lq;
end

== matlab function Final/B2B Rig /Motor PMSM/Torque Calculation ==
  data: id_m input; Te_motor output; iq_m input; Ld input; Lq input; lambda_m input; p input
function Te_motor = fcn(id_m,iq_m,Ld,Lq,lambda_m,p)

Te_motor = 1.5*p*(lambda_m*iq_m + (Ld - Lq)*id_m*iq_m);
